simulink model "sl_driveline"  (R2015a)
settings: Solver=ode45  StartTime=0.0  StopTime=15.0  RelTol=1e-3
InitFcn:
  | if ~exist('x0')
  |   x0 = [5 5 0];
  |   msgbox(sprintf('x0 not defined in workspace, setting it to [%g %g %g]\n', x0));
  | end
  | if ~exist('L')
  |   L = [1 -2 4];
  |   msgbox(sprintf('L not defined in workspace, setting it to [%g %g %g]\n', L));
  | end
  | % clean up old vehicle icons
  | set(0, 'ShowHiddenHandles', 'on')
  | delete(findobj('Tag', 'vehicle'))
  | set(0, 'ShowHiddenHandles', 'off')
StopFcn:
  | % update the XY scope
  | set(0, 'ShowHiddenHandles', 'on')
  | fig = findobj('name', 'XY');
  | ax = findobj(fig, 'type', 'axes');
  | axes(ax)
  | grid on
  | hold on
  | plot_vehicle(x0, 'r', 'Tag', 'vehicle')
  | plot_homline(L, 'r--', 'Tag', 'vehicle')
  | hold off
  | set(0, 'ShowHiddenHandles', 'off')
libraries: roblocks x2, simulink x1
settings Model: Creator=pic  LastModifiedBy=corkep
settings SolverCC: ZeroCrossAlgorithm=Adaptive
settings DataIOCC: LimitDataPoints=off  ReturnWorkspaceOutputs=on  TimeSaveName=t  OutputSaveName=y
settings OptimizationCC: ExpressionDepthLimit=2147483647
settings DebuggingCC: UnderspecifiedInitializationDetection=Classic  MergeDetectMultiDrivingBlocksExec=none  SolverPrmCheckMsg=warning  StateNameClashWarn=warning
settings GRTTargetCC: CombineOutputUpdateFcns=off  GRTInterface=on

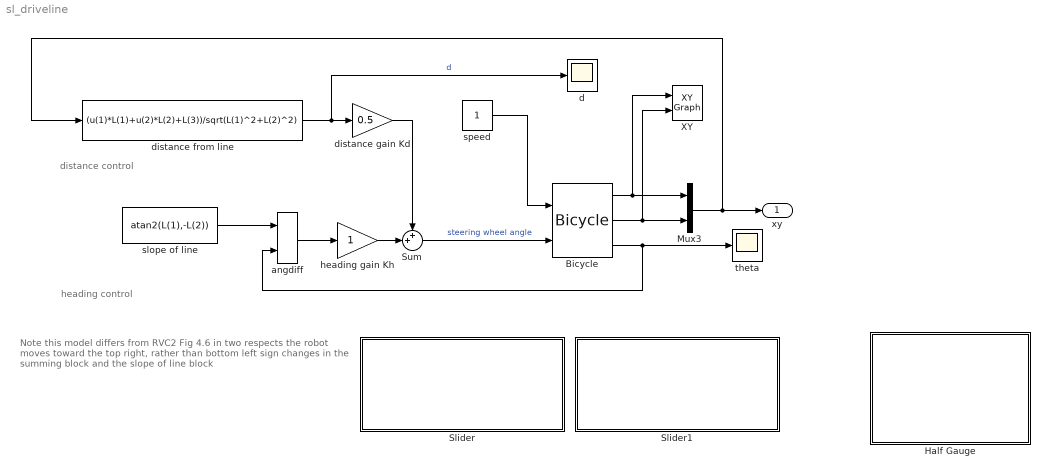
== system sl_driveline ==
  note: Note this model differs from RVC2 Fig 4.6 in two respects
      | the robot moves toward the top right, rather than bottom left
      | sign changes in the summing block and the slope of line block
  note: distance control
  note: heading control
  Bicycle : roblocks/Vehicles/Bicycle  vlim=1  accel=1  alim=1  steer_rate=Inf  L=1  x0=x0
  Half Gauge : Subsystem  DialogController=hmiCreateDDGDialog  IsWebBlock=on  mask(MathWorksWebBlock){webBlockId=6fa49c64-ed8a-4855-a04f-4b44e314a076, webBlockType=semicirculargauge, ShowInLibBrowser=on, ShowInitialText=on, HMISrcModelName=sl_driveline}
      mask prompts: webBlockId "WebBlock Id"; webBlockType "WebBlock Type"; HMISrcModelName "Source Model"
      mask help: Display an input value on a semicircular scale.
      mask Help: helpview([docroot '/mapfiles/simulink.map'], 'hmi_half_gauge')
      mask Display:
      | if strcmp(get_param(bdroot(gcb),'BlockDiagramType'),'library')
      |  image([(matlabroot) '/toolbox/simulink/hmi/icons/SemiCircularGauge.png'])
      | end
  Mux3 : Mux  Inputs=2
  Slider : Subsystem  Description=Replaced Block  mask(Replaced Block){}
      mask help: This block has been replaced with an empty subsystem because it used functionality that is unavailable in Simulink R2015a.
      mask Display: fprintf('Replaced: %s\n','Dashboard Widget')
  Slider1 : Subsystem  Description=Replaced Block  mask(Replaced Block){}
      mask help: This block has been replaced with an empty subsystem because it used functionality that is unavailable in Simulink R2015a.
      mask Display: fprintf('Replaced: %s\n','Dashboard Widget')
  Sum : Sum  Inputs=++|
  XY : simulink/Sinks/XY Graph  xmin=-10  xmax=10  ymin=-10  ymax=10  st=-1
  angdiff : roblocks/Toolbox/angdiff
  d : Scope
      settings: TimeRange=auto  MaxDataPoints=5000  SaveToWorkspace=off  YMin=-4.54438  YMax=0.65016  SampleTime=-1
  distance from line : Fcn  Expr=(u(1)*L(1)+u(2)*L(2)+L(3))/sqrt(L(1)^2+L(2)^2)
  distance gain Kd : Gain  Gain=0.5
  heading gain Kh : Gain
  slope of line : Constant  Value=atan2(L(1),-L(2))
  speed : Constant  VectorParams1D=off  SampleTime=0.02
  theta : Scope
      settings: TimeRange=auto  MaxDataPoints=5000  SaveToWorkspace=off  SaveName=ScopeData  YMin=-1.13424  YMax=0.68802  SampleTime=-1
  xy : Outport
  wires:
  Mux3/1 -> distance from line/1, xy/1
  slope of line/1 -> angdiff/1
  angdiff/1 -> heading gain Kh/1
  heading gain Kh/1 -> Sum/2
  speed/1 -> Bicycle/1
  Sum/1 -> Bicycle/2  "steering wheel angle"
  distance from line/1 -> distance gain Kd/1, d/1  "d"
  Bicycle/1 -> XY/1, Mux3/1
  Bicycle/2 -> XY/2, Mux3/2
  Bicycle/3 -> angdiff/2, theta/1
  distance gain Kd/1 -> Sum/1

== system sl_driveline/Half Gauge ==

== system sl_driveline/Slider ==

== system sl_driveline/Slider1 ==
